simulink library "marine_hydro"  (R2019b)
settings: Solver=ode45  StartTime=0.0  StopTime=10.0  RelTol=1e-3
undefined symbols (not defined in the file): Hoerner, magnitude, slcm, vessel, vesselABC
libraries: simulink x60, marine_gnc x22, $bdroot x9
(part 2 of 4)

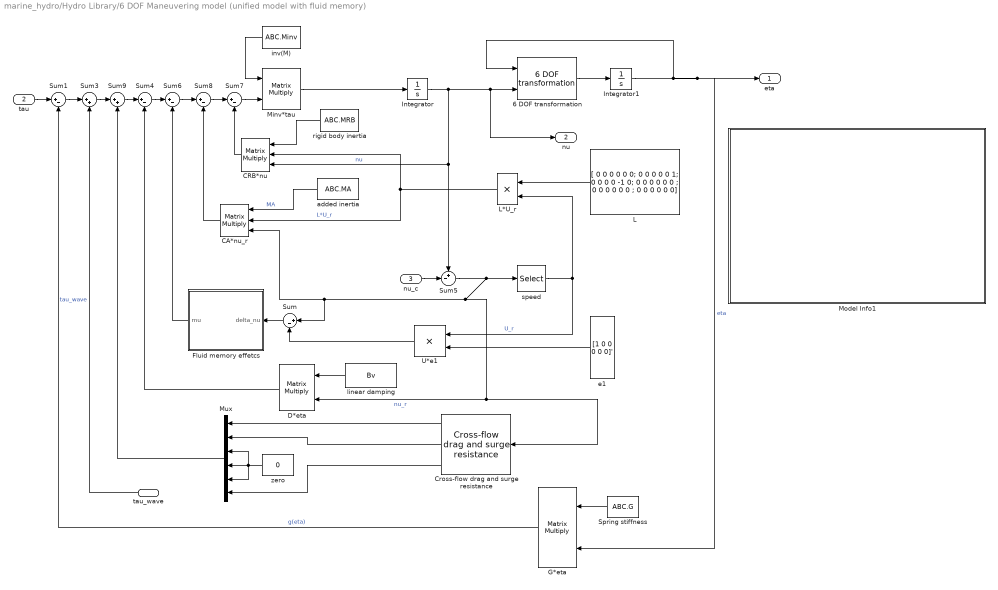
== system marine_hydro/Hydro Library/6 DOF Maneuvering model (unified model with fluid memory) ==
  tau_wave : Inport
  tau : Inport  Port=2
  nu_c : Inport  Port=3
  6 DOF transformation : marine_gnc/Models/ Kinematics/6 DOF transformation  SystemSampleTime=-1
  CA*nu_r : Product  Inputs=3  Multiplication=Matrix(*)  RndMeth=Zero
  CRB*nu : Product  Inputs=3  Multiplication=Matrix(*)  RndMeth=Zero
  Cross-flow drag and surge resistance : $bdroot/Hydro Library/Cross-flow drag and surge resistance  SystemSampleTime=-1  N=20  Lpp=vessel.main.Lpp  CD=CY_2D  Cx=CX  Ax=Axc  Ay=Ayc  rho_w=rho
  "D*eta " : Product  Multiplication=Matrix(*)  SaturateOnIntegerOverflow=on  OutDataTypeStr=Inherit: Same as first input
  Fluid memory effetcs : Subsystem
  G*eta : Product  Multiplication=Matrix(*)  SaturateOnIntegerOverflow=on  OutDataTypeStr=Inherit: Same as first input
  Integrator : Integrator
  Integrator1 : Integrator
  L : Constant  Value=|
      | [ 0     0     0     0     0     0;   0     0     0     0     0     1;
      |      0     0     0     0    -1     0;	
      |      0     0     0     0     0     0	;
      |      0     0     0     0     0     0	
      | ;     0     0     0     0     0     0]
  L*U_r : Product  RndMeth=Zero
  Minv*tau : Product  Inputs=**  Multiplication=Matrix(*)  SaturateOnIntegerOverflow=on  OutDataTypeStr=Inherit: Same as first input
  Model Info1 : Subsystem  LoadFcn=slcm LoadBlock;  InitFcn=slcm('UpdateAllCMBlocksInThisModelInit')  mask(CMBlock){InitialSaveTempField=, InitialBlockCM=None, BlockCM=None, Frame=on, SaveTempField=, DisplayStringWithTags=|, MaskDisplayString=This is an example block based on Perez and Fossen (2007).\nThe model includes speed-dependent fluid memory effects \ncross-flow drag and surge resistance (quadratic drag).\nYou must inlcude maneuvering coefficients your self. \n\nAlso notice that viscous roll damping is computed under the assumption \nof zero speed. Forward speed effects can, however, be added if necessary.\n\nReference\nT. Perez and T. I. Fossen (2007). Kinematic Models for Seakeeping\nand Maneuvering of Marine Vessels. Modeling, Identification\nand Control, MIC-28(1):1-12.\n\nDownload link: www.marinecontrol.org\n\nAuthor: Thor I. Fossen\nThu Sep 17 11:19:48 2009, HorizontalTextAlignment=Left, LeftAlignmentValue=0.02, SourceBlockDiagram=marine_hydro, TagMaxNumber=20, CMTag1=, CMTag2=, CMTag3=, CMTag4=, CMTag5=, CMTag6=, CMTag7=, CMTag8=, CMTag9=, CMTag10=, CMTag11=, CMTag12=, CMTag13=, CMTag14=, CMTag15=, CMTag16=, CMTag17=, CMTag18=, CMTag19=, CMTag20=}
      mask DisplayStringWithTags=|
      | This is an example block based on Perez and Fossen (2007).\nThe model includes speed-dependent fluid memory effects
      | cross-flow drag and surge resistance (quadratic drag).\nYou must inlcude maneuvering coefficients your self. \n
      | Also notice that viscous roll damping is computed under the assumption \nof zero speed. Forward speed effects can, however, be added if necessary.
      |
      | Reference
      | T. Perez and T. I. Fossen (2007). Kinematic Models for Seakeeping
      | and Maneuvering of Marine Vessels. Modeling, Identification\nand Control, MIC-28(1):1-12.\n
      | Download link: www.marinecontrol.org
      |
      | Author: Thor I. Fossen
      | %<LastModificationDate>
      mask help: This block allows revision control information to be displayed within the model.
      settings: CopyFcn=slcm CopyBlock;  DeleteFcn=slcm Cancel;  PostSaveFcn=slcm('UpdateAllCMBlocksInThisModel')  NameChangeFcn=slcm Rename;  OpenFcn=slcm
      mask Display: text(str2num(LeftAlignmentValue), 0.5, MaskDisplayString, 'HorizontalAlignment', HorizontalTextAlignment)
  Mux : Mux  Inputs=6
  Spring stiffness : Constant  Value=ABC.G
  Sum : Sum  Inputs=|+-
  Sum{1,4,6..8} (5 alike) : Sum  Inputs=|+-  SaturateOnIntegerOverflow=on
  Sum3 : Sum  Inputs=|++  SaturateOnIntegerOverflow=on
  Sum5 : Sum  Inputs=+-|  SaturateOnIntegerOverflow=on
  Sum9 : Sum  Inputs=|++  SaturateOnIntegerOverflow=on
  U*e1 : Product  RndMeth=Zero
  added inertia : Constant  Value=ABC.MA
  e1 : Constant  Value=[1 0 0 0 0 0]'  VectorParams1D=off
  inv(M) : Constant  Value=ABC.Minv
  linear damping : Constant  Value=Bv
  rigid body inertia : Constant  Value=ABC.MRB
  speed : Selector  InputPortWidth=6  IndexOptions=Index vector (dialog)  Indices=[1]  OutputSizes=1
  zero : Constant  Value=0
  eta : Outport
  nu : Outport  Port=2
  wires:
  speed/1 -> L*U_r/2, U*e1/1  "U_r"
  inv(M)/1 -> Minv*tau/1
  e1/1 -> U*e1/2
  U*e1/1 -> Sum/2
  Sum/1 -> Fluid memory effetcs/1(delta_nu)
  L*U_r/1 -> CA*nu_r/2, CRB*nu/2  "L*U_r"
  L/1 -> L*U_r/1
  Mux/1 -> Sum9/2
  Sum9/1 -> Sum4/1
  zero/1 -> Mux/5, Mux/3, Mux/4
  Cross-flow drag and surge resistance/3 -> Mux/6
  Cross-flow drag and surge resistance/2 -> Mux/2
  Cross-flow drag and surge resistance/1 -> Mux/1
  CA*nu_r/1 -> Sum8/2
  Sum8/1 -> Sum7/1
  CRB*nu/1 -> Sum7/2
  Fluid memory effetcs/1(mu) -> Sum6/2
  Sum7/1 -> Minv*tau/2
  Sum5/1 -> speed/1, Sum/1, CA*nu_r/3, Cross-flow drag and surge resistance/1, "D*eta "/2  "nu_r"
  nu_c/1 -> Sum5/2
  "D*eta "/1 -> Sum4/2
  linear damping/1 -> "D*eta "/1
  Integrator/1 -> CRB*nu/3, Sum5/1, nu/1, 6 DOF transformation/2  "nu"
  Sum1/1 -> Sum3/1
  Spring stiffness/1 -> G*eta/1
  added inertia/1 -> CA*nu_r/1  "MA"
  6 DOF transformation/1 -> Integrator1/1
  Integrator1/1 -> G*eta/2, eta/1, 6 DOF transformation/1  "eta"
  G*eta/1 -> Sum1/2  "g(eta)"
  rigid body inertia/1 -> CRB*nu/1
  tau/1 -> Sum1/1
  tau_wave/1 -> Sum3/2  "tau_wave"
  Sum3/1 -> Sum9/1
  Sum6/1 -> Sum8/1
  Sum4/1 -> Sum6/1
  Minv*tau/1 -> Integrator/1

== system marine_hydro/Hydro Library/Cross-flow drag and surge resistance ==
  nu_r : Inport
  "2D drag coefficient " : Constant  Value=CD
  Abs1 : Abs  SaturateOnIntegerOverflow=on
  Cross-flow drag trapezoidal integration : Subsystem  TreatAsAtomicUnit=on
  Drag coefficient : Constant  Value=Cx
  Frontal area : Constant  Value=Ax
  Gain : Gain  Gain=-0.5  SaturateOnIntegerOverflow=on  OutDataTypeStr=Inherit: Same as input  ParamDataTypeStr=Inherit: Same as input
  Gain1 : Gain  Gain=-0.5  SaturateOnIntegerOverflow=on  OutDataTypeStr=Inherit: Same as input  ParamDataTypeStr=Inherit: Same as input
  Gain2 : Gain  Gain=0.5  SaturateOnIntegerOverflow=on  OutDataTypeStr=Inherit: Same as input  ParamDataTypeStr=Inherit: Same as input
  Gain3 : Gain  Gain=-1  SaturateOnIntegerOverflow=on  OutDataTypeStr=Inherit: Same as input  ParamDataTypeStr=Inherit: Same as input
  Lpp : Constant  Value=Lpp
  N : Constant  Value=N
  Product5 : Product  Inputs=3  SaturateOnIntegerOverflow=on  OutDataTypeStr=Inherit: Same as first input
  Product7 : Product  SaturateOnIntegerOverflow=on  OutDataTypeStr=Inherit: Same as first input
  Product8 : Product  SaturateOnIntegerOverflow=on  OutDataTypeStr=Inherit: Same as first input
  Selector : Selector  InputPortWidth=6  IndexOptions=Index vector (dialog)  Indices=[2]  OutputSizes=1
  Selector1 : Selector  InputPortWidth=6  IndexOptions=Index vector (dialog)  Indices=[6]  OutputSizes=1
  Selector2 : Selector  InputPortWidth=6  IndexOptions=Index vector (dialog)  Indices=[1]  OutputSizes=1
  Sum : Sum  Inputs=+-|  SaturateOnIntegerOverflow=on  InputSameDT=on  OutDataTypeStr=Inherit: Same as first input
  Transversal area/Lpp : Constant  Value=Ay/Lpp
  constant : Constant
  dx : Product  Inputs=/*  RndMeth=Zero
  dx1 : Product  Inputs=4  RndMeth=Zero
  dx2 : Product  Inputs=4  RndMeth=Zero
  rho : Constant  Value=rho_w
  X_drag : Outport
  Y_drag : Outport  Port=2
  N_drag : Outport  Port=3
  wires:
  Product5/1 -> Product8/2
  Product7/1 -> Product8/1
  Abs1/1 -> Product7/1
  Selector2/1 -> Abs1/1, Product7/2  "u_r"
  Frontal area/1 -> Gain2/1
  Gain2/1 -> Product5/1
  "2D drag coefficient "/1 -> dx2/4, dx1/4
  Transversal area/Lpp/1 -> dx2/3, dx1/3
  N/1 -> Sum/1, Cross-flow drag trapezoidal integration/1(N)  "N"
  Sum/1 -> dx/1  "N-1"
  dx/1 -> Cross-flow drag trapezoidal integration/2(dx)
  constant/1 -> Sum/2
  Lpp/1 -> dx/2
  Selector1/1 -> Cross-flow drag trapezoidal integration/4(r)  "r"
  Selector/1 -> Cross-flow drag trapezoidal integration/3(v_r)  "v_r"
  Cross-flow drag trapezoidal integration/2(sum2) -> Gain/1
  Cross-flow drag trapezoidal integration/1(sum1) -> Gain1/1
  Gain3/1 -> X_drag/1
  Product8/1 -> Gain3/1
  nu_r/1 -> Selector2/1, Selector/1, Selector1/1
  Gain1/1 -> dx1/1
  dx1/1 -> Y_drag/1
  Gain/1 -> dx2/1
  dx2/1 -> N_drag/1
  rho/1 -> dx1/2, dx2/2, Product5/3
  Drag coefficient/1 -> Product5/2

== system marine_hydro/Hydro Library/Motion RAO (U=0) ==
  eta LF : Inport
  Waves : Inport  Port=2
  6DOF rotation matrix in yaw : Subsystem
  Bus Selector : BusSelector  OutputSignals=Psi,Wavenum,Omega,Phase,Zeta_a
  Clock : Clock
  Output smoothing : Subsystem
  Position phase : marine_gnc/Models/Environmental Loads/Utilities/Position phase  SystemSampleTime=-1
  Product1 : Product  Inputs=**  SaturateOnIntegerOverflow=on  OutDataTypeStr=Inherit: Same as first input
  Sum : Sum  Inputs=-++  SaturateOnIntegerOverflow=on
  Wave component loop : Subsystem  TreatAsAtomicUnit=on
  Width : Width  DataType=int32
  Yaw quantizer : marine_gnc/Models/Environmental Loads/Utilities/Yaw quantizer  SystemSampleTime=-1  quant_flag=RAO_yaw_quantization_flag  quant=RAO_yaw_quant  back=RAO_yaw_back
  "[-inf inf] to [-pi pi]" : marine_gnc/Utilities/Math Operations/[-inf inf] to [-pi pi]  SystemSampleTime=-1
  yaw angle : Selector  InputPortWidth=6  IndexOptions=Index vector (dialog)  Indices=6  OutputSizes=1
  eta WF : Outport
  nu WF : Outport  Port=2
  nu_dot WF : Outport  Port=3
  wires:
  Position phase/1 -> Sum/1
  "[-inf inf] to [-pi pi]"/1 -> Wave component loop/2(Psi_r)
  Yaw quantizer/1 -> "[-inf inf] to [-pi pi]"/1
  Wave component loop/3(nu_dot WF) -> Output smoothing/3("nu_dot WF ")
  Wave component loop/2(nu WF) -> Output smoothing/2("nu WF ")
  Width/1 -> Wave component loop/1(number of iterations)
  Bus Selector/5 -> Wave component loop/5(Zeta_a)  "<Zeta_a>"
  Sum/1 -> Wave component loop/4(Phase_tot)  "Phase_tot"
  6DOF rotation matrix in yaw/1(R(psi)*V) -> eta WF/1
  Bus Selector/3 -> Product1/1, Wave component loop/3(Omega), Width/1  "<Omega>"
  yaw angle/1 -> Yaw quantizer/1, 6DOF rotation matrix in yaw/1(psi)
  Clock/1 -> Product1/2
  Bus Selector/1 -> Yaw quantizer/2, Position phase/1  "<Psi>"
  Product1/1 -> Sum/2
  Waves/1 -> Bus Selector/1
  Bus Selector/4 -> Sum/3  "<Phase>"
  Bus Selector/2 -> Position phase/2  "<Wavenum>"
  eta LF/1 -> Position phase/3, yaw angle/1
  Output smoothing/2(nu WF) -> nu WF/1
  Output smoothing/3(nu_dot WF) -> nu_dot WF/1
  Wave component loop/1(eta_h WF) -> Output smoothing/1(eta_h WF)
  Wave component loop/4(nu_dot rate) -> Output smoothing/4(nu_dot rate)
  Output smoothing/1("eta_h WF ") -> 6DOF rotation matrix in yaw/2(V)

== system marine_hydro/Hydro Library/WD for heading1 ==
  psi : Inport
  psi_wave : Inport  Port=2
  Omega : Inport  Port=3
  Zeta_a : Inport  Port=4
  U : Inport  Port=5
  Sum1 : Sum  Inputs=-+|
  Wave component loop : Subsystem  TreatAsAtomicUnit=on
  Width : Width  DataType=int32
  tau_WD : Outport
  wires:
  psi/1 -> Sum1/1  "psi"
  U/1 -> Wave component loop/5(U)
  Wave component loop/1(tau_WD) -> tau_WD/1
  Sum1/1 -> Wave component loop/2(Psi_r)
  Zeta_a/1 -> Wave component loop/4(Zeta_a)
  Omega/1 -> Width/1, Wave component loop/3(Omega)
  psi_wave/1 -> Sum1/2
  Width/1 -> Wave component loop/1(number of iterations)

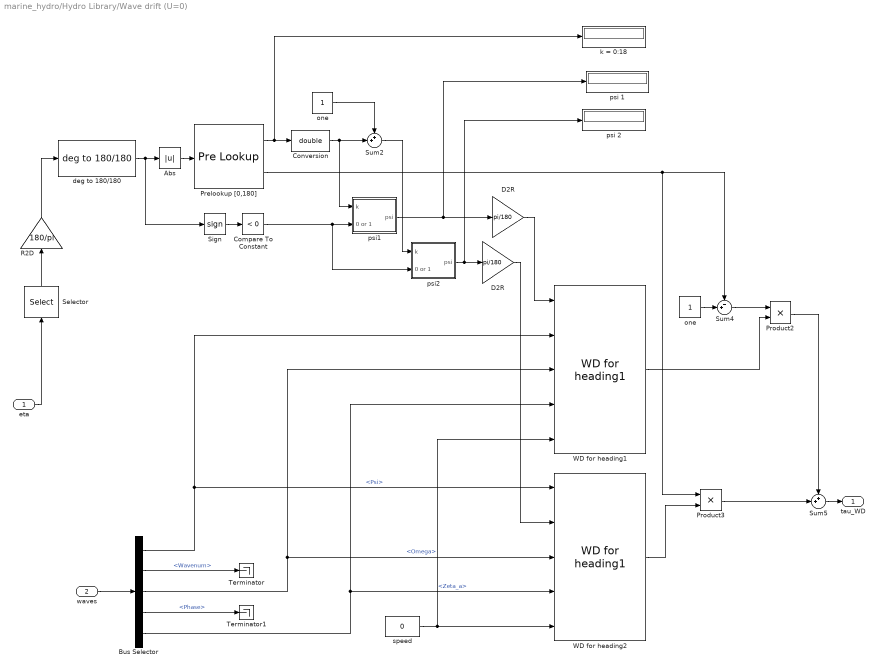
== system marine_hydro/Hydro Library/Wave drift (U=0) ==
  eta : Inport
  waves : Inport  Port=2
  Abs : Abs  SaturateOnIntegerOverflow=on
  Bus Selector : BusSelector  OutputSignals=Psi,Wavenum,Omega,Phase,Zeta_a
  Compare To Constant : simulink/Logic and Bit Operations/Compare To Constant  SystemSampleTime=-1  relop=<  const=0  LogicOutDataTypeMode=uint8  ZeroCross=off
  Conversion : DataTypeConversion  OutDataTypeStr=double
  D2R : Gain  Gain=pi/180
  "D2R " : Gain  Gain=pi/180
  Prelookup [0,180] : PreLookup  BreakpointsData=[0:10:180]  IndexSearchMethod=Evenly spaced points  BeginIndexSearchUsingPreviousIndexResult=on
  Product2 : Product  RndMeth=Zero
  Product3 : Product  RndMeth=Zero
  R2D : Gain  Gain=180/pi
  Selector : Selector  InputPortWidth=6  IndexOptions=Index vector (dialog)  Indices=[6]  OutputSizes=1
  Sign : Signum
  Sum2 : Sum  Inputs=++|
  Sum4 : Sum  Inputs=-+|
  Sum5 : Sum  Inputs=++|
  Terminator : Terminator
  Terminator1 : Terminator
  WD for heading1 : $bdroot/Hydro Library/WD for heading1  SystemSampleTime=-1  ForceRAO_Freq=vessel.forceRAO.w  WD_Freq=vessel.driftfrc.w  RAO_Vel=vessel.velocities  ForceRAO_Amp=vessel.forceRAO.amp  ForceRAO_Phase=vessel.forceRAO.phase  WD_Amp=vessel.driftfrc.amp  RAO_add_omega_0=on  RAO_add_omega_inf=on
  WD for heading2 : $bdroot/Hydro Library/WD for heading1  SystemSampleTime=-1  ForceRAO_Freq=vessel.forceRAO.w  WD_Freq=vessel.driftfrc.w  RAO_Vel=vessel.velocities  ForceRAO_Amp=vessel.forceRAO.amp  ForceRAO_Phase=vessel.forceRAO.phase  WD_Amp=vessel.driftfrc.amp  RAO_add_omega_0=on  RAO_add_omega_inf=on
  deg to 180/180 : marine_gnc/Utilities/Math Operations/deg to 180//180  SystemSampleTime=-1
  k = 0:18 : Display
  one : Constant
  "one " : Constant
  psi 1 : Display
  psi 2 : Display
  psi1 : Subsystem
  psi2 : Subsystem
  speed : Constant  Value=0
  tau_WD : Outport
  wires:
  "D2R "/1 -> WD for heading2/2
  D2R/1 -> WD for heading1/1
  Bus Selector/4 -> Terminator1/1  "<Phase>"
  Bus Selector/1 -> WD for heading2/1, WD for heading1/2  "<Psi>"
  Bus Selector/2 -> Terminator/1  "<Wavenum>"
  Bus Selector/5 -> WD for heading1/4, WD for heading2/4  "<Zeta_a>"
  Bus Selector/3 -> WD for heading1/3, WD for heading2/3  "<Omega>"
  speed/1 -> WD for heading1/5, WD for heading2/5
  R2D/1 -> deg to 180/180/1
  Selector/1 -> R2D/1
  Sum5/1 -> tau_WD/1
  waves/1 -> Bus Selector/1
  psi2/1(psi) -> psi 2/1, "D2R "/1
  Conversion/1 -> psi1/1(k), Sum2/2
  Prelookup [0,180]/2 -> Sum4/1, Product3/1
  psi1/1(psi) -> psi 1/1, D2R/1
  Compare To Constant/1 -> psi2/2(0 or 1), psi1/2(0 or 1)
  Sign/1 -> Compare To Constant/1
  Abs/1 -> Prelookup [0,180]/1
  deg to 180/180/1 -> Sign/1, Abs/1
  Sum2/1 -> psi2/1(k)
  one/1 -> Sum2/1
  Prelookup [0,180]/1 -> k = 0:18/1, Conversion/1
  Product2/1 -> Sum5/1
  Product3/1 -> Sum5/2
  WD for heading1/1 -> Product2/2
  Sum4/1 -> Product2/1
  "one "/1 -> Sum4/2
  eta/1 -> Selector/1
  WD for heading2/1 -> Product3/2

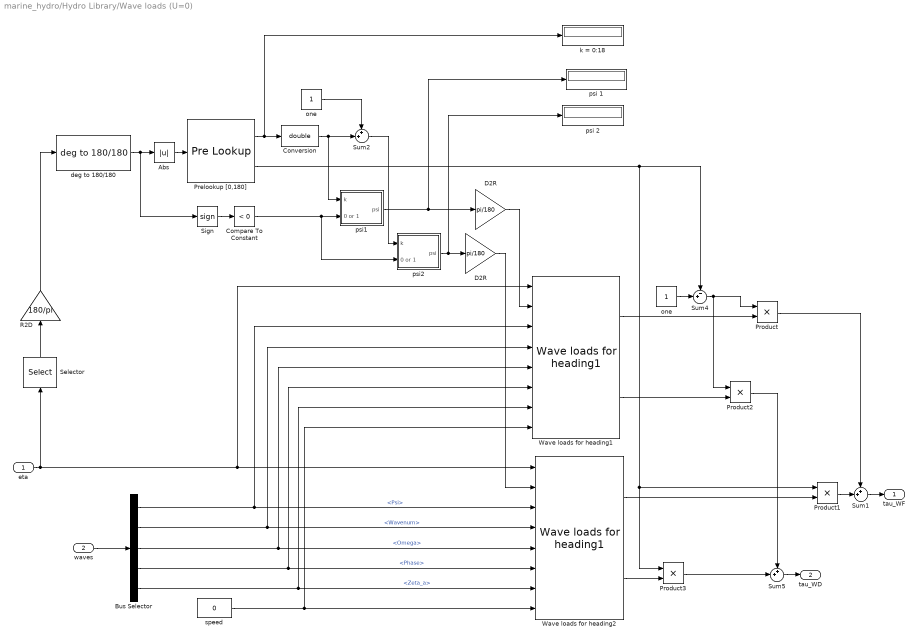
== system marine_hydro/Hydro Library/Wave loads (U=0) ==
  eta : Inport
  waves : Inport  Port=2
  Abs : Abs  SaturateOnIntegerOverflow=on
  Bus Selector : BusSelector  OutputSignals=Psi,Wavenum,Omega,Phase,Zeta_a
  Compare To Constant : simulink/Logic and Bit Operations/Compare To Constant  SystemSampleTime=-1  relop=<  const=0  LogicOutDataTypeMode=uint8  ZeroCross=off
  Conversion : DataTypeConversion  OutDataTypeStr=double
  D2R : Gain  Gain=pi/180
  "D2R " : Gain  Gain=pi/180
  Prelookup [0,180] : PreLookup  BreakpointsData=[0:10:180]  IndexSearchMethod=Evenly spaced points  BeginIndexSearchUsingPreviousIndexResult=on
  Product{,1..3} (4 alike) : Product  RndMeth=Zero
  R2D : Gain  Gain=180/pi
  Selector : Selector  InputPortWidth=6  IndexOptions=Index vector (dialog)  Indices=[6]  OutputSizes=1
  Sign : Signum
  Sum1 : Sum  Inputs=++|
  Sum2 : Sum  Inputs=++|
  Sum4 : Sum  Inputs=-+|
  Sum5 : Sum  Inputs=++|
  Wave loads for heading1 : $bdroot/Hydro Library/Wave loads for heading1  SystemSampleTime=-1  ForceRAO_Freq=vessel.forceRAO.w  WD_Freq=vessel.driftfrc.w  RAO_Vel=vessel.velocities  ForceRAO_Amp=vessel.forceRAO.amp  ForceRAO_Phase=vessel.forceRAO.phase  WD_Amp=vessel.driftfrc.amp  RAO_add_omega_0=on  RAO_add_omega_inf=on
  Wave loads for heading2 : $bdroot/Hydro Library/Wave loads for heading1  SystemSampleTime=-1  ForceRAO_Freq=vessel.forceRAO.w  WD_Freq=vessel.driftfrc.w  RAO_Vel=vessel.velocities  ForceRAO_Amp=vessel.forceRAO.amp  ForceRAO_Phase=vessel.forceRAO.phase  WD_Amp=vessel.driftfrc.amp  RAO_add_omega_0=on  RAO_add_omega_inf=on
  deg to 180/180 : marine_gnc/Utilities/Math Operations/deg to 180//180  SystemSampleTime=-1
  k = 0:18 : Display
  one : Constant
  "one " : Constant
  psi 1 : Display
  psi 2 : Display
  psi1 : Subsystem
  psi2 : Subsystem
  speed : Constant  Value=0
  tau_WF : Outport
  tau_WD : Outport  Port=2
  wires:
  speed/1 -> Wave loads for heading1/8, Wave loads for heading2/8
  Wave loads for heading2/1 -> Product1/2
  Wave loads for heading2/2 -> Product3/2
  eta/1 -> Wave loads for heading1/1, Wave loads for heading2/1, Selector/1
  Bus Selector/1 -> Wave loads for heading1/3, Wave loads for heading2/3  "<Psi>"
  Bus Selector/2 -> Wave loads for heading1/4, Wave loads for heading2/4  "<Wavenum>"
  Bus Selector/3 -> Wave loads for heading1/5, Wave loads for heading2/5  "<Omega>"
  Bus Selector/4 -> Wave loads for heading1/6, Wave loads for heading2/6  "<Phase>"
  Bus Selector/5 -> Wave loads for heading1/7, Wave loads for heading2/7  "<Zeta_a>"
  Wave loads for heading1/1 -> Product/2
  Product/1 -> Sum1/1
  Product1/1 -> Sum1/2
  "one "/1 -> Sum4/2
  Sum4/1 -> Product/1, Product2/1
  Wave loads for heading1/2 -> Product2/2
  Product3/1 -> Sum5/2
  Product2/1 -> Sum5/1
  Prelookup [0,180]/1 -> Conversion/1, k = 0:18/1
  one/1 -> Sum2/1
  Sum2/1 -> psi2/1(k)
  deg to 180/180/1 -> Abs/1, Sign/1
  Abs/1 -> Prelookup [0,180]/1
  Sign/1 -> Compare To Constant/1
  Compare To Constant/1 -> psi1/2(0 or 1), psi2/2(0 or 1)
  psi1/1(psi) -> D2R/1, psi 1/1
  Prelookup [0,180]/2 -> Product3/1, Product1/1, Sum4/1
  Conversion/1 -> Sum2/2, psi1/1(k)
  psi2/1(psi) -> "D2R "/1, psi 2/1
  D2R/1 -> Wave loads for heading1/2
  "D2R "/1 -> Wave loads for heading2/2
  Sum1/1 -> tau_WF/1
  waves/1 -> Bus Selector/1
  Sum5/1 -> tau_WD/1
  Selector/1 -> R2D/1
  R2D/1 -> deg to 180/180/1

== system marine_hydro/Hydro Library/Wave loads (U>0) ==
  eta : Inport
  waves : Inport  Port=2
  U : Inport  Port=3
  Abs : Abs  SaturateOnIntegerOverflow=on
  Conversion : DataTypeConversion  OutDataTypeStr=double
  Prelookup : PreLookup  BreakpointsData=vessel.velocities  IndexSearchMethod=Linear search  BeginIndexSearchUsingPreviousIndexResult=on
  Product{,1..3} (4 alike) : Product  RndMeth=Zero
  Sum1 : Sum  Inputs=++|
  Sum2 : Sum  Inputs=++|
  Sum4 : Sum  Inputs=-+|
  Sum5 : Sum  Inputs=++|
  Wave loads U = U1 : Subsystem
  Wave loads U = U2 : Subsystem
  one : Constant
  "one " : Constant
  tau_WF : Outport
  tau_WD : Outport  Port=2
  wires:
  waves/1 -> Wave loads U = U1/2(waves), Wave loads U = U2/2(waves)
  eta/1 -> Wave loads U = U1/1(eta), Wave loads U = U2/1(eta)
  Conversion/1 -> Sum2/2, Wave loads U = U1/3(U_idx)
  Abs/1 -> Prelookup/1
  one/1 -> Sum2/1
  Prelookup/1 -> Conversion/1
  Sum2/1 -> Wave loads U = U2/3(U_idx)
  Sum5/1 -> tau_WD/1
  Sum1/1 -> tau_WF/1
  Prelookup/2 -> Sum4/1, Product1/1, Product3/1
  Product2/1 -> Sum5/1
  Product3/1 -> Sum5/2
  Sum4/1 -> Product2/1, Product/1
  "one "/1 -> Sum4/2
  Product1/1 -> Sum1/2
  Product/1 -> Sum1/1
  Wave loads U = U1/1(tau_WF) -> Product/2
  Wave loads U = U2/2(tau_WD) -> Product3/2
  Wave loads U = U2/1(tau_WF) -> Product1/2
  Wave loads U = U1/2(tau_WD) -> Product2/2
  U/1 -> Abs/1

== system marine_hydro/Hydro Library/Wave loads for heading1 ==
  eta : Inport
  psi : Inport  Port=2
  psi_wave : Inport  Port=3
  wavenum : Inport  Port=4
  Omega : Inport  Port=5
  Phase : Inport  Port=6
  Zeta_a : Inport  Port=7
  U : Inport  Port=8
  Clock : Clock
  Position phase : marine_gnc/Models/Environmental Loads/Utilities/Position phase  SystemSampleTime=-1
  Product1 : Product  Inputs=**  SaturateOnIntegerOverflow=on  OutDataTypeStr=Inherit: Same as first input
  Sum : Sum  Inputs=-++  SaturateOnIntegerOverflow=on
  Sum1 : Sum  Inputs=-+|
  Wave component loop : Subsystem  TreatAsAtomicUnit=on
  Width : Width  DataType=int32
  tau_WF : Outport
  tau_WD : Outport  Port=2
  wires:
  Position phase/1 -> Sum/1
  Width/1 -> Wave component loop/1(number of iterations)
  Sum/1 -> Wave component loop/4(Phase_tot)  "Phase_tot"
  Clock/1 -> Product1/2
  Product1/1 -> Sum/2
  Wave component loop/1(tau_WF) -> tau_WF/1
  eta/1 -> Position phase/3
  psi_wave/1 -> Position phase/1, Sum1/2
  wavenum/1 -> Position phase/2
  Omega/1 -> Product1/1, Wave component loop/3(Omega), Width/1
  Phase/1 -> Sum/3
  Zeta_a/1 -> Wave component loop/5(Zeta_a)
  Sum1/1 -> Wave component loop/2(Psi_r)
  Wave component loop/2(tau_WD) -> tau_WD/1
  U/1 -> Wave component loop/6(U)
  psi/1 -> Sum1/1  "psi"

== system marine_hydro/Hydro Library/zero speed viiscous roll damping ==
  p : Inport
  A44 : Constant  Value=vesselABC.A44(:,:,1)
  B44 : Constant  Value=vesselABC.B44(:,:,1)
  B44_inf : Constant  Value=vesselABC.B44_inf(1)
  C44 : Constant  Value=vesselABC.C44(:,:,1)
  D44 : Constant  Value=vesselABC.D44(:,:,1)
  Integrator : Integrator
  Math Function : Math  Operator=transpose  SaturateOnIntegerOverflow=on
  Product{,1..2,4} (4 alike) : Product  Multiplication=Matrix(*)  RndMeth=Zero
  Product3 : Product  RndMeth=Zero
  Sum : Sum  Inputs=++|
  Sum1 : Sum  Inputs=|++
  Sum2 : Sum  Inputs=++|
  K_visc : Outport
  wires:
  Product4/1 -> Sum2/1
  B44_inf/1 -> Product4/1
  Sum2/1 -> K_visc/1
  p/1 -> Product4/2, Product1/2, Product3/2
  Integrator/1 -> Product/2, Product2/2
  A44/1 -> Product/1
  Product1/1 -> Sum/1
  Product/1 -> Sum/2
  Sum/1 -> Integrator/1
  C44/1 -> Math Function/1
  D44/1 -> Product3/1
  Product3/1 -> Sum1/2
  Product2/1 -> Sum1/1
  Sum1/1 -> Sum2/2
  B44/1 -> Product1/1
  Math Function/1 -> Product2/1

== system marine_hydro/Vessel Templates/DP Force RAO model - zero speed ==
  Gain : Gain  SaturateOnIntegerOverflow=on  OutDataTypeStr=Inherit: Same as input  ParamDataTypeStr=Inherit: Same as input

== system marine_hydro/Vessel Templates/DP Motion RAO model - zero speed ==
  Gain : Gain  SaturateOnIntegerOverflow=on  OutDataTypeStr=Inherit: Same as input  ParamDataTypeStr=Inherit: Same as input

== system marine_hydro/Vessel Templates/Maneuvering Force RAO model - forward speed ==
  Gain : Gain  SaturateOnIntegerOverflow=on  OutDataTypeStr=Inherit: Same as input  ParamDataTypeStr=Inherit: Same as input

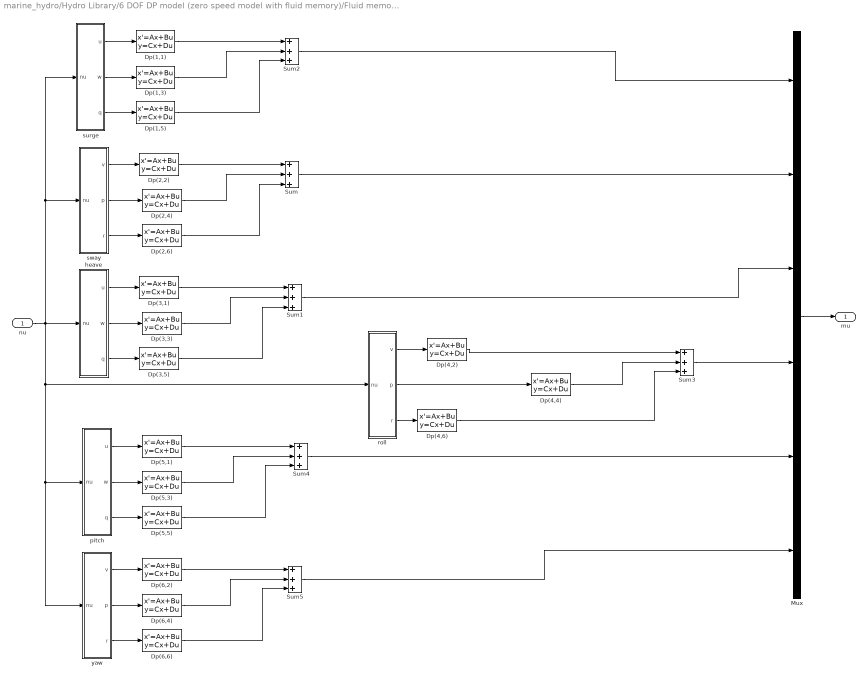
== system marine_hydro/Hydro Library/6 DOF DP model (zero speed model with fluid memory)/Fluid memory effetcs ==
  nu : Inport
  Dp(1,1) : StateSpace  A=ABC.Ar{1,1}  B=ABC.Br{1,1}  C=ABC.Cr{1,1}  D=ABC.Dr{1,1}  InitialCondition=0
  Dp(1,3) : StateSpace  A=ABC.Ar{1,3}  B=ABC.Br{1,3}  C=ABC.Cr{1,3}  D=ABC.Dr{1,3}  InitialCondition=0
  Dp(1,5) : StateSpace  A=ABC.Ar{1,5}  B=ABC.Br{1,5}  C=ABC.Cr{1,5}  D=ABC.Dr{1,5}  InitialCondition=0
  Dp(2,2) : StateSpace  A=ABC.Ar{2,2}  B=ABC.Br{2,2}  C=ABC.Cr{2,2}  D=ABC.Dr{2,2}  InitialCondition=0
  Dp(2,4) : StateSpace  A=ABC.Ar{2,4}  B=ABC.Br{2,4}  C=ABC.Cr{2,4}  D=ABC.Dr{2,4}  InitialCondition=0
  Dp(2,6) : StateSpace  A=ABC.Ar{2,6}  B=ABC.Br{2,6}  C=ABC.Cr{2,6}  D=ABC.Dr{2,6}  InitialCondition=0
  Dp(3,1) : StateSpace  A=ABC.Ar{3,1}  B=ABC.Br{3,1}  C=ABC.Cr{3,1}  D=ABC.Dr{3,1}  InitialCondition=0
  Dp(3,3) : StateSpace  A=ABC.Ar{3,3}  B=ABC.Br{3,3}  C=ABC.Cr{3,3}  D=ABC.Dr{3,3}  InitialCondition=0
  Dp(3,5) : StateSpace  A=ABC.Ar{3,5}  B=ABC.Br{3,5}  C=ABC.Cr{3,5}  D=ABC.Dr{3,5}  InitialCondition=0
  Dp(4,2) : StateSpace  A=ABC.Ar{4,2}  B=ABC.Br{4,2}  C=ABC.Cr{4,2}  D=ABC.Dr{4,2}  InitialCondition=0
  Dp(4,4) : StateSpace  A=ABC.Ar{4,4}  B=ABC.Br{4,4}  C=ABC.Cr{4,4}  D=ABC.Dr{4,4}  InitialCondition=0
  Dp(4,6) : StateSpace  A=ABC.Ar{4,6}  B=ABC.Br{4,6}  C=ABC.Cr{4,6}  D=ABC.Dr{4,6}  InitialCondition=0
  Dp(5,1) : StateSpace  A=ABC.Ar{5,1}  B=ABC.Br{5,1}  C=ABC.Cr{5,1}  D=ABC.Dr{5,1}  InitialCondition=0
  Dp(5,3) : StateSpace  A=ABC.Ar{5,3}  B=ABC.Br{5,3}  C=ABC.Cr{5,3}  D=ABC.Dr{5,3}  InitialCondition=0
  Dp(5,5) : StateSpace  A=ABC.Ar{5,5}  B=ABC.Br{5,5}  C=ABC.Cr{5,5}  D=ABC.Dr{5,5}  InitialCondition=0
  Dp(6,2) : StateSpace  A=ABC.Ar{6,2}  B=ABC.Br{6,2}  C=ABC.Cr{6,2}  D=ABC.Dr{6,2}  InitialCondition=0
  Dp(6,4) : StateSpace  A=ABC.Ar{6,4}  B=ABC.Br{6,4}  C=ABC.Cr{6,4}  D=ABC.Dr{6,4}  InitialCondition=0
  Dp(6,6) : StateSpace  A=ABC.Ar{6,6}  B=ABC.Br{6,6}  C=ABC.Cr{6,6}  D=ABC.Dr{6,6}  InitialCondition=0
  Mux : Mux  Inputs=6
  Sum{,1..5} (6 alike) : Sum  Inputs=+++  SaturateOnIntegerOverflow=on
  heave : Subsystem
  pitch : Subsystem
  roll : Subsystem
  surge : Subsystem
  sway : Subsystem
  yaw : Subsystem
  mu : Outport
  wires:
  Sum4/1 -> Mux/5
  Dp(2,2)/1 -> Sum/1
  Dp(2,4)/1 -> Sum/2
  Dp(2,6)/1 -> Sum/3
  Sum/1 -> Mux/2
  sway/1(v) -> Dp(2,2)/1
  sway/2(p) -> Dp(2,4)/1
  sway/3(r) -> Dp(2,6)/1
  Dp(3,3)/1 -> Sum1/2
  Dp(3,5)/1 -> Sum1/3
  Sum1/1 -> Mux/3
  heave/3(q) -> Dp(3,5)/1
  heave/2(w) -> Dp(3,3)/1
  heave/1(u) -> Dp(3,1)/1
  Dp(3,1)/1 -> Sum1/1
  nu/1 -> heave/1(nu), sway/1(nu), surge/1(nu), roll/1(nu), pitch/1(nu), yaw/1(nu)
  Mux/1 -> mu/1
  Dp(1,3)/1 -> Sum2/2
  Dp(1,5)/1 -> Sum2/3
  Sum2/1 -> Mux/1
  surge/3(q) -> Dp(1,5)/1
  surge/2(w) -> Dp(1,3)/1
  surge/1(u) -> Dp(1,1)/1
  Dp(1,1)/1 -> Sum2/1
  Dp(4,2)/1 -> Sum3/1
  Dp(4,6)/1 -> Sum3/3
  roll/1(v) -> Dp(4,2)/1
  roll/3(r) -> Dp(4,6)/1
  Dp(5,3)/1 -> Sum4/2
  Dp(5,5)/1 -> Sum4/3
  pitch/3(q) -> Dp(5,5)/1
  pitch/2(w) -> Dp(5,3)/1
  pitch/1(u) -> Dp(5,1)/1
  Dp(5,1)/1 -> Sum4/1
  Sum3/1 -> Mux/4
  Dp(6,2)/1 -> Sum5/1
  Dp(6,4)/1 -> Sum5/2
  Dp(6,6)/1 -> Sum5/3
  yaw/1(v) -> Dp(6,2)/1
  yaw/2(p) -> Dp(6,4)/1
  yaw/3(r) -> Dp(6,6)/1
  Sum5/1 -> Mux/6
  roll/2(p) -> Dp(4,4)/1
  Dp(4,4)/1 -> Sum3/2

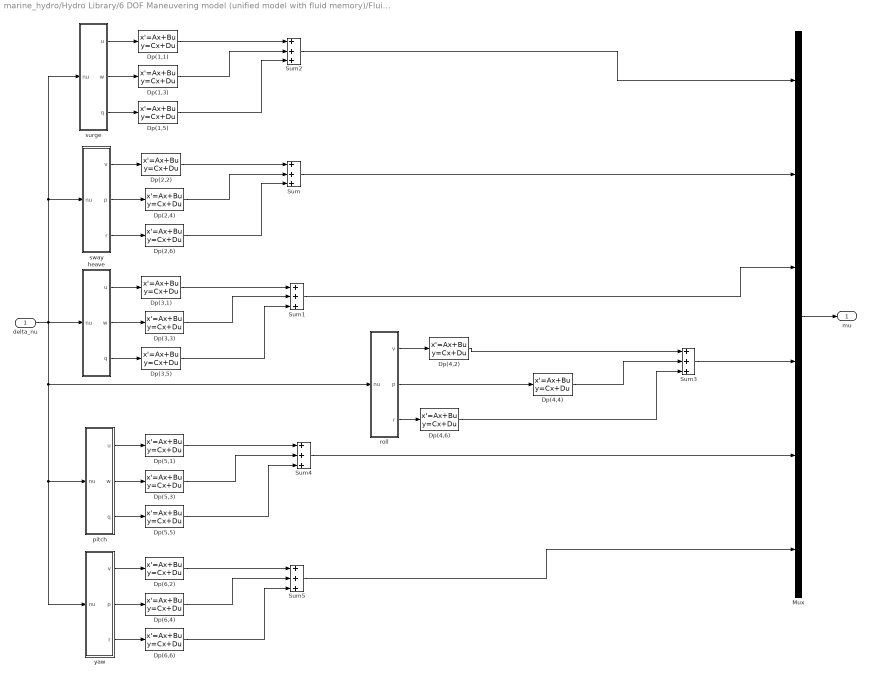
== system marine_hydro/Hydro Library/6 DOF Maneuvering model (unified model with fluid memory)/Fluid memory effetcs ==
  delta_nu : Inport
  Dp(1,1) : StateSpace  A=ABC.Ar{1,1}  B=ABC.Br{1,1}  C=ABC.Cr{1,1}  D=ABC.Dr{1,1}  InitialCondition=0
  Dp(1,3) : StateSpace  A=ABC.Ar{1,3}  B=ABC.Br{1,3}  C=ABC.Cr{1,3}  D=ABC.Dr{1,3}  InitialCondition=0
  Dp(1,5) : StateSpace  A=ABC.Ar{1,5}  B=ABC.Br{1,5}  C=ABC.Cr{1,5}  D=ABC.Dr{1,5}  InitialCondition=0
  Dp(2,2) : StateSpace  A=ABC.Ar{2,2}  B=ABC.Br{2,2}  C=ABC.Cr{2,2}  D=ABC.Dr{2,2}  InitialCondition=0
  Dp(2,4) : StateSpace  A=ABC.Ar{2,4}  B=ABC.Br{2,4}  C=ABC.Cr{2,4}  D=ABC.Dr{2,4}  InitialCondition=0
  Dp(2,6) : StateSpace  A=ABC.Ar{2,6}  B=ABC.Br{2,6}  C=ABC.Cr{2,6}  D=ABC.Dr{2,6}  InitialCondition=0
  Dp(3,1) : StateSpace  A=ABC.Ar{3,1}  B=ABC.Br{3,1}  C=ABC.Cr{3,1}  D=ABC.Dr{3,1}  InitialCondition=0
  Dp(3,3) : StateSpace  A=ABC.Ar{3,3}  B=ABC.Br{3,3}  C=ABC.Cr{3,3}  D=ABC.Dr{3,3}  InitialCondition=0
  Dp(3,5) : StateSpace  A=ABC.Ar{3,5}  B=ABC.Br{3,5}  C=ABC.Cr{3,5}  D=ABC.Dr{3,5}  InitialCondition=0
  Dp(4,2) : StateSpace  A=ABC.Ar{4,2}  B=ABC.Br{4,2}  C=ABC.Cr{4,2}  D=ABC.Dr{4,2}  InitialCondition=0
  Dp(4,4) : StateSpace  A=ABC.Ar{4,4}  B=ABC.Br{4,4}  C=ABC.Cr{4,4}  D=ABC.Dr{4,4}  InitialCondition=0
  Dp(4,6) : StateSpace  A=ABC.Ar{4,6}  B=ABC.Br{4,6}  C=ABC.Cr{4,6}  D=ABC.Dr{4,6}  InitialCondition=0
  Dp(5,1) : StateSpace  A=ABC.Ar{5,1}  B=ABC.Br{5,1}  C=ABC.Cr{5,1}  D=ABC.Dr{5,1}  InitialCondition=0
  Dp(5,3) : StateSpace  A=ABC.Ar{5,3}  B=ABC.Br{5,3}  C=ABC.Cr{5,3}  D=ABC.Dr{5,3}  InitialCondition=0
  Dp(5,5) : StateSpace  A=ABC.Ar{5,5}  B=ABC.Br{5,5}  C=ABC.Cr{5,5}  D=ABC.Dr{5,5}  InitialCondition=0
  Dp(6,2) : StateSpace  A=ABC.Ar{6,2}  B=ABC.Br{6,2}  C=ABC.Cr{6,2}  D=ABC.Dr{6,2}  InitialCondition=0
  Dp(6,4) : StateSpace  A=ABC.Ar{6,4}  B=ABC.Br{6,4}  C=ABC.Cr{6,4}  D=ABC.Dr{6,4}  InitialCondition=0
  Dp(6,6) : StateSpace  A=ABC.Ar{6,6}  B=ABC.Br{6,6}  C=ABC.Cr{6,6}  D=ABC.Dr{6,6}  InitialCondition=0
  Mux : Mux  Inputs=6
  Sum{,1..5} (6 alike) : Sum  Inputs=+++  SaturateOnIntegerOverflow=on
  heave : Subsystem
  pitch : Subsystem
  roll : Subsystem
  surge : Subsystem
  sway : Subsystem
  yaw : Subsystem
  mu : Outport
  wires:
  Sum4/1 -> Mux/5
  Dp(2,2)/1 -> Sum/1
  Dp(2,4)/1 -> Sum/2
  Dp(2,6)/1 -> Sum/3
  Sum/1 -> Mux/2
  sway/1(v) -> Dp(2,2)/1
  sway/2(p) -> Dp(2,4)/1
  sway/3(r) -> Dp(2,6)/1
  Dp(3,3)/1 -> Sum1/2
  Dp(3,5)/1 -> Sum1/3
  Sum1/1 -> Mux/3
  heave/3(q) -> Dp(3,5)/1
  heave/2(w) -> Dp(3,3)/1
  heave/1(u) -> Dp(3,1)/1
  Dp(3,1)/1 -> Sum1/1
  delta_nu/1 -> heave/1(nu), sway/1(nu), surge/1(nu), roll/1(nu), pitch/1(nu), yaw/1(nu)
  Mux/1 -> mu/1
  Dp(1,3)/1 -> Sum2/2
  Dp(1,5)/1 -> Sum2/3
  Sum2/1 -> Mux/1
  surge/3(q) -> Dp(1,5)/1
  surge/2(w) -> Dp(1,3)/1
  surge/1(u) -> Dp(1,1)/1
  Dp(1,1)/1 -> Sum2/1
  Dp(4,2)/1 -> Sum3/1
  Dp(4,6)/1 -> Sum3/3
  roll/1(v) -> Dp(4,2)/1
  roll/3(r) -> Dp(4,6)/1
  Dp(5,3)/1 -> Sum4/2
  Dp(5,5)/1 -> Sum4/3
  pitch/3(q) -> Dp(5,5)/1
  pitch/2(w) -> Dp(5,3)/1
  pitch/1(u) -> Dp(5,1)/1
  Dp(5,1)/1 -> Sum4/1
  Sum3/1 -> Mux/4
  Dp(6,2)/1 -> Sum5/1
  Dp(6,4)/1 -> Sum5/2
  Dp(6,6)/1 -> Sum5/3
  yaw/1(v) -> Dp(6,2)/1
  yaw/2(p) -> Dp(6,4)/1
  yaw/3(r) -> Dp(6,6)/1
  Sum5/1 -> Mux/6
  roll/2(p) -> Dp(4,4)/1
  Dp(4,4)/1 -> Sum3/2

== system marine_hydro/Hydro Library/6 DOF Maneuvering model (unified model with fluid memory)/Model Info1 ==
  EmptySubsystem : Subsystem

== system marine_hydro/Hydro Library/Cross-flow drag and surge resistance/Cross-flow drag trapezoidal integration ==
  N : Inport
  dx : Inport  Port=2
  v_r : Inport  Port=3
  r : Inport  Port=4
  Abs : Abs  SaturateOnIntegerOverflow=on
  For Iterator : ForIterator  ResetStates=reset  IterationSource=external  IterationVariableDataType=double
  If i=1 or i=N : If  NumInputs=2  IfExpression=u1 == 1 | u1 == u2
  Lpp/2 : Constant  Value=Lpp/2
  Merge : Merge
  Product : Product  Inputs=**  SaturateOnIntegerOverflow=on  OutDataTypeStr=Inherit: Same as first input
  Product1 : Product  Inputs=**  SaturateOnIntegerOverflow=on  OutDataTypeStr=Inherit: Same as first input
  Product3 : Product  SaturateOnIntegerOverflow=on  OutDataTypeStr=Inherit: Same as first input
  Product4 : Product  SaturateOnIntegerOverflow=on  OutDataTypeStr=Inherit: Same as first input
  Sum : Sum  Inputs=|++  SaturateOnIntegerOverflow=on  InputSameDT=on  OutDataTypeStr=Inherit: Same as first input
  Sum1 : Sum  Inputs=++|  SaturateOnIntegerOverflow=on
  Sum2 : Sum  Inputs=|++  SaturateOnIntegerOverflow=on  InputSameDT=on  OutDataTypeStr=Inherit: Same as first input
  Sum3 : Sum  Inputs=+-|  SaturateOnIntegerOverflow=on  InputSameDT=on  OutDataTypeStr=Inherit: Same as first input
  Sum4 : Sum  Inputs=+-|  SaturateOnIntegerOverflow=on  InputSameDT=on  OutDataTypeStr=Inherit: Same as first input
  constant : Constant
  memory1 : Memory  InheritSampleTime=on
  memory2 : Memory  InheritSampleTime=on
  multiply with 0.5 : Subsystem  TreatAsAtomicUnit=on
  multiply with 1 : Subsystem  TreatAsAtomicUnit=on
  x * r : Product  SaturateOnIntegerOverflow=on  OutDataTypeStr=Inherit: Same as first input
  sum1 : Outport
  sum2 : Outport  Port=2
  wires:
  Merge/1 -> Product4/1, Sum/2
  multiply with 1/1(Out1) -> Merge/2
  multiply with 0.5/1(Out1) -> Merge/1
  If i=1 or i=N/2 -> multiply with 1/Action
  If i=1 or i=N/1 -> multiply with 0.5/Action
  Product/1 -> multiply with 0.5/1(In1), multiply with 1/1(In1)
  Product3/1 -> Product/2
  Product4/1 -> Sum2/2
  r/1 -> x * r/1
  Sum3/1 -> Product4/2, x * r/2  "x"
  constant/1 -> Sum4/2
  Sum4/1 -> Product1/2  "i-1"
  Product1/1 -> Sum3/1
  Lpp/2/1 -> Sum3/2
  dx/1 -> Product/1, Product1/1  "dx"
  memory2/1 -> Sum2/1
  Sum2/1 -> memory2/1, sum2/1
  memory1/1 -> Sum/1
  Sum/1 -> memory1/1, sum1/1
  v_r/1 -> Sum1/1
  Abs/1 -> Product3/1
  x * r/1 -> Sum1/2
  Sum1/1 -> Abs/1, Product3/2
  N/1 -> If i=1 or i=N/2, For Iterator/1
  For Iterator/1 -> Sum4/1, If i=1 or i=N/1  "i"

== system marine_hydro/Hydro Library/Motion RAO (U=0)/6DOF rotation matrix in yaw ==
  psi : Inport
  V : Inport  Port=2
  Mux1 : Mux  Inputs=2
  Rotation matrix in yaw : marine_gnc/Models/ Kinematics/Rotation matrix in yaw   SystemSampleTime=-1
  Selector : Selector  InputPortWidth=6  IndexOptions=Index vector (dialog)  Indices=[4 5 6]  OutputSizes=1
  Selector2 : Selector  InputPortWidth=6  IndexOptions=Index vector (dialog)  Indices=[1 2 3]  OutputSizes=1
  R(psi)*V : Outport
  wires:
  Selector/1 -> Mux1/2
  Mux1/1 -> R(psi)*V/1
  Selector2/1 -> Rotation matrix in yaw/2
  psi/1 -> Rotation matrix in yaw/1
  V/1 -> Selector2/1, Selector/1
  Rotation matrix in yaw/1 -> Mux1/1

== system marine_hydro/Hydro Library/Motion RAO (U=0)/Output smoothing ==
  eta_h WF : Inport
  "nu WF " : Inport  Port=2
  "nu_dot WF " : Inport  Port=3
  nu_dot rate : Inport  Port=4
  Output smoothing flag : Constant  Value=RAO_smoothing_flag
  Signal smoothing : marine_gnc/Models/Environmental Loads/Utilities/Signal smoothing  SystemSampleTime=-1
  Signal smoothing1 : marine_gnc/Models/Environmental Loads/Utilities/Signal smoothing  SystemSampleTime=-1
  Signal smoothing2 : marine_gnc/Models/Environmental Loads/Utilities/Signal smoothing  SystemSampleTime=-1
  Switch1 : Switch  Threshold=0.5
  Switch2 : Switch  Threshold=0.5
  Switch3 : Switch  Threshold=0.5
  "eta_h WF " : Outport
  nu WF : Outport  Port=2
  nu_dot WF : Outport  Port=3
  wires:
  Output smoothing flag/1 -> Switch2/2, Switch1/2, Switch3/2
  Signal smoothing/1 -> Switch2/1
  eta_h WF/1 -> Signal smoothing/1, Switch2/3
  "nu WF "/1 -> Signal smoothing1/1, Signal smoothing/2, Switch1/3
  Signal smoothing1/1 -> Switch1/1
  Switch2/1 -> "eta_h WF "/1
  "nu_dot WF "/1 -> Signal smoothing2/1, Signal smoothing1/2, Switch3/3
  Signal smoothing2/1 -> Switch3/1
  nu_dot rate/1 -> Signal smoothing2/2
  Switch3/1 -> nu_dot WF/1
  Switch1/1 -> nu WF/1

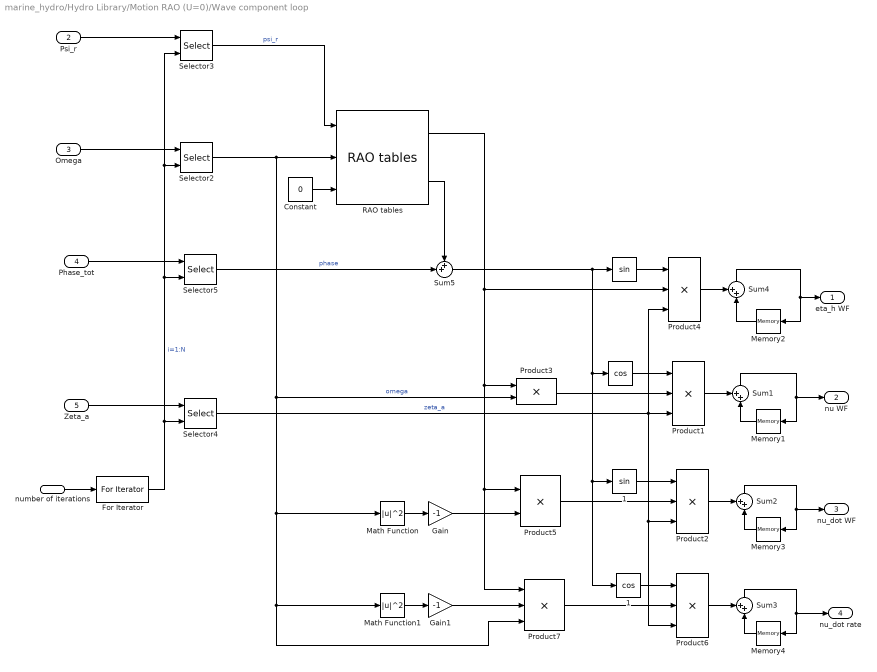
== system marine_hydro/Hydro Library/Motion RAO (U=0)/Wave component loop ==
  number of iterations : Inport
  Psi_r : Inport  Port=2
  Omega : Inport  Port=3
  Phase_tot : Inport  Port=4
  Zeta_a : Inport  Port=5
  "              " : Trigonometry  Operator=cos
  "                " : Trigonometry
  "                1" : Trigonometry
  "              1" : Trigonometry  Operator=cos
  Constant : Constant  Value=0
  For Iterator : ForIterator  ResetStates=reset  IterationSource=external  IterationVariableDataType=double
  Gain : Gain  Gain=-1  SaturateOnIntegerOverflow=on  OutDataTypeStr=Inherit: Same as input  ParamDataTypeStr=Inherit: Same as input
  Gain1 : Gain  Gain=-1  SaturateOnIntegerOverflow=on  OutDataTypeStr=Inherit: Same as input  ParamDataTypeStr=Inherit: Same as input
  Math Function : Math  Operator=magnitude^2  SaturateOnIntegerOverflow=on
  Math Function1 : Math  Operator=magnitude^2  SaturateOnIntegerOverflow=on
  Memory{1..4} (4 alike) : Memory  InitialCondition=[0 0 0 0 0 0]'  InheritSampleTime=on
  Product{1..2,4,6} (4 alike) : Product  Inputs=3  SaturateOnIntegerOverflow=on  OutDataTypeStr=Inherit: Same as first input
  Product3 : Product  Inputs=**  SaturateOnIntegerOverflow=on  OutDataTypeStr=Inherit: Same as first input
  Product5 : Product  Inputs=**  SaturateOnIntegerOverflow=on  OutDataTypeStr=Inherit: Same as first input
  Product7 : Product  Inputs=***  SaturateOnIntegerOverflow=on  OutDataTypeStr=Inherit: Same as first input
  RAO tables : marine_gnc/Models/Environmental Loads/Utilities/RAO tables  SystemSampleTime=-1  RAO_Freq=RAO_Freq  RAO_Dir=RAO_Dir  RAO_Vel=RAO_Vel  RAO_Amp=RAO_Amp  RAO_Phase=RAO_Phase
  Selector{2..5} (4 alike) : Selector  IndexOptions=Index vector (port)  Indices=[1 3]  OutputSizes=1
  Sum{1..5} (5 alike) : Sum  Inputs=++|  SaturateOnIntegerOverflow=on
  eta_h WF : Outport
  nu WF : Outport  Port=2
  nu_dot WF : Outport  Port=3
  nu_dot rate : Outport  Port=4
  wires:
  Product3/1 -> Product1/2
  Product5/1 -> Product2/2
  Gain/1 -> Product5/2
  Math Function/1 -> Gain/1
  "                1"/1 -> Product2/1
  Sum2/1 -> Memory3/1, nu_dot WF/1
  Product2/1 -> Sum2/1
  Memory3/1 -> Sum2/2
  Product1/1 -> Sum1/1
  Sum1/1 -> Memory1/1, nu WF/1
  Memory1/1 -> Sum1/2
  "              "/1 -> Product1/1
  Selector4/1 -> Product4/3, Product1/3, Product2/3, Product6/3  "zeta_a"
  "                "/1 -> Product4/1
  Sum5/1 -> "              "/1, "                1"/1, "              1"/1, "                "/1
  Zeta_a/1 -> Selector4/1
  Phase_tot/1 -> Selector5/1
  RAO tables/2 -> Sum5/1
  RAO tables/1 -> Product3/1, Product5/1, Product7/1, Product4/2
  Constant/1 -> RAO tables/3
  Psi_r/1 -> Selector3/1
  For Iterator/1 -> Selector4/2, Selector5/2, Selector2/2, Selector3/2  "i=1:N"
  Omega/1 -> Selector2/1
  number of iterations/1 -> For Iterator/1
  Sum4/1 -> Memory2/1, eta_h WF/1
  Memory2/1 -> Sum4/2
  Product4/1 -> Sum4/1
  Selector5/1 -> Sum5/2  "phase"
  Selector2/1 -> RAO tables/2, Product3/2, Math Function/1, Math Function1/1, Product7/3  "omega"
  Selector3/1 -> RAO tables/1  "psi_r"
  Sum3/1 -> nu_dot rate/1, Memory4/1
  Product6/1 -> Sum3/1
  Memory4/1 -> Sum3/2
  Gain1/1 -> Product7/2
  Math Function1/1 -> Gain1/1
  "              1"/1 -> Product6/1
  Product7/1 -> Product6/2

== system marine_hydro/Hydro Library/WD for heading1/Wave component loop ==
  number of iterations : Inport
  Psi_r : Inport  Port=2
  Omega : Inport  Port=3
  Zeta_a : Inport  Port=4
  U : Inport  Port=5
  Direct Lookup Table (n-D) Beta : simulink/Lookup Tables/Direct Lookup Table (n-D)  maskTabDims=1  explicitNumDims=1  outDims=Element  tabIsInput=off  mxTable=vessel.headings  clipFlag=Warning  samptime=-1
      settings: SourceProductName=Simulink  SourceProductBaseCode=SL
  Direct Lookup Table (n-D) Velocity : simulink/Lookup Tables/Direct Lookup Table (n-D)  maskTabDims=1  explicitNumDims=1  outDims=Element  tabIsInput=off  mxTable=RAO_Vel  clipFlag=Warning  samptime=-1
      settings: SourceProductName=Simulink  SourceProductBaseCode=SL
  For Iterator : ForIterator  ResetStates=reset  IterationSource=external  IterationVariableDataType=double
  Memory1 : Memory  InitialCondition=[0 0 0 0 0 0]'  InheritSampleTime=on
  Prelookup1 : PreLookup  BreakpointsData=vessel.headings  OutputSelection=Index only  IndexSearchMethod=Evenly spaced points  BeginIndexSearchUsingPreviousIndexResult=on
  Prelookup2 : PreLookup  BreakpointsData=RAO_Vel  OutputSelection=Index only  IndexSearchMethod=Linear search  BeginIndexSearchUsingPreviousIndexResult=on
  Product3 : Product  Inputs=3  SaturateOnIntegerOverflow=on  OutDataTypeStr=Inherit: Same as first input
  Selector2 : Selector  IndexOptions=Index vector (port)  Indices=[1 3]  OutputSizes=1
  Selector3 : Selector  IndexOptions=Index vector (port)  Indices=[1 3]  OutputSizes=1
  Selector4 : Selector  IndexOptions=Index vector (port)  Indices=[1 3]  OutputSizes=1
  Sum1 : Sum  Inputs=++|  SaturateOnIntegerOverflow=on
  WD RAO tables : Subsystem  mask(RAO table lookup){}
      mask help:
      | Perform 3D table lookup in 6DOF RAO amplitudes and phases, using the relative wave heading psi_r, wave frequency omega and vessel velocity vel as inputs. See documentation of the Motion RAO block or Force RAO block for details. A warning is issued if the input is outside the range spanned by the RAOs.
      |
      | Author: Oyvind N. Smogeli and Thor I. Fossen, 2005-05-03
  "[-inf inf] to [-pi pi]" : marine_gnc/Utilities/Math Operations/[-inf inf] to [-pi pi]  SystemSampleTime=-1
  "[-pi pi] to [0 2pi]" : Subsystem  mask([-inf inf] to [-pi pi]){}
      mask help: Converts an angle in rad to (-pi pi)
  tau_WD : Outport
  wires:
  WD RAO tables/1(amp) -> Product3/1
  Direct Lookup Table (n-D) Velocity/1 -> WD RAO tables/3(U)
  Prelookup2/1 -> Direct Lookup Table (n-D) Velocity/1
  Direct Lookup Table (n-D) Beta/1 -> WD RAO tables/1(beta)
  Prelookup1/1 -> Direct Lookup Table (n-D) Beta/1
  "[-inf inf] to [-pi pi]"/1 -> "[-pi pi] to [0 2pi]"/1(x [-pi pi])
  For Iterator/1 -> Selector2/2, Selector4/2, Selector3/2  "i=1:N"
  Selector2/1 -> WD RAO tables/2(w)  "omega"
  "[-pi pi] to [0 2pi]"/1(0<y<2pi) -> Prelookup1/1
  Product3/1 -> Sum1/1
  Memory1/1 -> Sum1/2
  Sum1/1 -> tau_WD/1, Memory1/1
  Selector3/1 -> "[-inf inf] to [-pi pi]"/1  "psi_r"
  number of iterations/1 -> For Iterator/1
  Omega/1 -> Selector2/1
  Psi_r/1 -> Selector3/1
  U/1 -> Prelookup2/1
  Zeta_a/1 -> Selector4/1
  Selector4/1 -> Product3/3, Product3/2  "zeta_a"

== system marine_hydro/Hydro Library/Wave drift (U=0)/psi1 ==
  k : Inport
  0 or 1 : Inport  Port=2
  Gain1 : Gain  Gain=20
  Gain2 : Gain  Gain=10
  Product : Product  RndMeth=Zero
  Sum7 : Sum  Inputs=-+|
  Sum8 : Sum  Inputs=++|
  const : Constant  Value=18
  psi : Outport
  wires:
  0 or 1/1 -> Product/2
  Sum8/1 -> psi/1
  k/1 -> Gain2/1, Sum7/1
  Gain2/1 -> Sum8/1
  Product/1 -> Sum8/2
  Gain1/1 -> Product/1
  Sum7/1 -> Gain1/1
  const/1 -> Sum7/2

== system marine_hydro/Hydro Library/Wave drift (U=0)/psi2 ==
  k : Inport
  0 or 1 : Inport  Port=2
  Gain1 : Gain  Gain=20
  Gain2 : Gain  Gain=10
  Product : Product  RndMeth=Zero
  Sum7 : Sum  Inputs=-+|
  Sum8 : Sum  Inputs=++|
  const : Constant  Value=18
  psi : Outport
  wires:
  0 or 1/1 -> Product/2
  Sum8/1 -> psi/1
  k/1 -> Gain2/1, Sum7/1
  Gain2/1 -> Sum8/1
  Product/1 -> Sum8/2
  Gain1/1 -> Product/1
  Sum7/1 -> Gain1/1
  const/1 -> Sum7/2

== system marine_hydro/Hydro Library/Wave loads (U=0)/psi1 ==
  k : Inport
  0 or 1 : Inport  Port=2
  Gain1 : Gain  Gain=20
  Gain2 : Gain  Gain=10
  Product : Product  RndMeth=Zero
  Sum7 : Sum  Inputs=-+|
  Sum8 : Sum  Inputs=++|
  const : Constant  Value=18
  psi : Outport
  wires:
  const/1 -> Sum7/2
  Sum7/1 -> Gain1/1
  Gain1/1 -> Product/1
  Product/1 -> Sum8/2
  Gain2/1 -> Sum8/1
  k/1 -> Sum7/1, Gain2/1
  Sum8/1 -> psi/1
  0 or 1/1 -> Product/2

== system marine_hydro/Hydro Library/Wave loads (U=0)/psi2 ==
  k : Inport
  0 or 1 : Inport  Port=2
  Gain1 : Gain  Gain=20
  Gain2 : Gain  Gain=10
  Product : Product  RndMeth=Zero
  Sum7 : Sum  Inputs=-+|
  Sum8 : Sum  Inputs=++|
  const : Constant  Value=18
  psi : Outport
  wires:
  const/1 -> Sum7/2
  Sum7/1 -> Gain1/1
  Gain1/1 -> Product/1
  Product/1 -> Sum8/2
  Gain2/1 -> Sum8/1
  k/1 -> Sum7/1, Gain2/1
  Sum8/1 -> psi/1
  0 or 1/1 -> Product/2

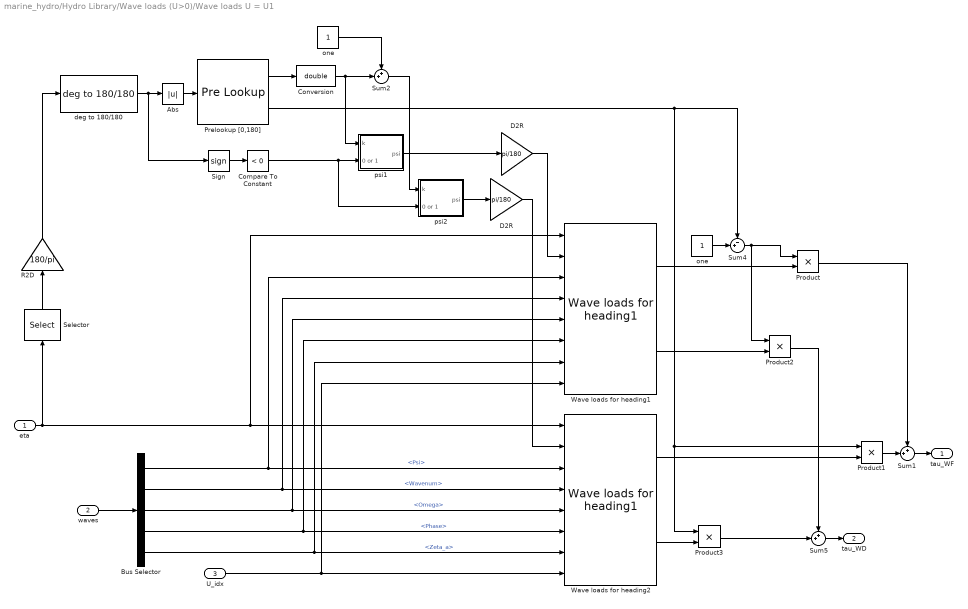
== system marine_hydro/Hydro Library/Wave loads (U>0)/Wave loads U = U1 ==
  eta : Inport
  waves : Inport  Port=2
  U_idx : Inport  Port=3
  Abs : Abs  SaturateOnIntegerOverflow=on
  Bus Selector : BusSelector  OutputSignals=Psi,Wavenum,Omega,Phase,Zeta_a
  Compare To Constant : simulink/Logic and Bit Operations/Compare To Constant  SystemSampleTime=-1  relop=<  const=0  LogicOutDataTypeMode=uint8  ZeroCross=off
  Conversion : DataTypeConversion  OutDataTypeStr=double
  D2R : Gain  Gain=pi/180
  "D2R " : Gain  Gain=pi/180
  Prelookup [0,180] : PreLookup  BreakpointsData=[0:10:180]  IndexSearchMethod=Evenly spaced points  BeginIndexSearchUsingPreviousIndexResult=on
  Product{,1..3} (4 alike) : Product  RndMeth=Zero
  R2D : Gain  Gain=180/pi
  Selector : Selector  InputPortWidth=6  IndexOptions=Index vector (dialog)  Indices=[6]  OutputSizes=1
  Sign : Signum
  Sum1 : Sum  Inputs=++|
  Sum2 : Sum  Inputs=++|
  Sum4 : Sum  Inputs=-+|
  Sum5 : Sum  Inputs=++|
  Wave loads for heading1 : $bdroot/Hydro Library/Wave loads for heading1  SystemSampleTime=-1  ForceRAO_Freq=vessel.forceRAO.w  WD_Freq=vessel.driftfrc.w  RAO_Vel=vessel.velocities  ForceRAO_Amp=vessel.forceRAO.amp  ForceRAO_Phase=vessel.forceRAO.phase  WD_Amp=vessel.driftfrc.amp  RAO_add_omega_0=on  RAO_add_omega_inf=on
  Wave loads for heading2 : $bdroot/Hydro Library/Wave loads for heading1  SystemSampleTime=-1  ForceRAO_Freq=vessel.forceRAO.w  WD_Freq=vessel.driftfrc.w  RAO_Vel=vessel.velocities  ForceRAO_Amp=vessel.forceRAO.amp  ForceRAO_Phase=vessel.forceRAO.phase  WD_Amp=vessel.driftfrc.amp  RAO_add_omega_0=on  RAO_add_omega_inf=on
  deg to 180/180 : marine_gnc/Utilities/Math Operations/deg to 180//180  SystemSampleTime=-1
  one : Constant
  "one " : Constant
  psi1 : Subsystem
  psi2 : Subsystem
  tau_WF : Outport
  tau_WD : Outport  Port=2
  wires:
  R2D/1 -> deg to 180/180/1
  Selector/1 -> R2D/1
  Sum5/1 -> tau_WD/1
  waves/1 -> Bus Selector/1
  Sum1/1 -> tau_WF/1
  "D2R "/1 -> Wave loads for heading2/2
  D2R/1 -> Wave loads for heading1/2
  psi2/1(psi) -> "D2R "/1
  Conversion/1 -> psi1/1(k), Sum2/2
  Prelookup [0,180]/2 -> Sum4/1, Product1/1, Product3/1
  psi1/1(psi) -> D2R/1
  Compare To Constant/1 -> psi2/2(0 or 1), psi1/2(0 or 1)
  Sign/1 -> Compare To Constant/1
  Abs/1 -> Prelookup [0,180]/1
  deg to 180/180/1 -> Sign/1, Abs/1
  Sum2/1 -> psi2/1(k)
  one/1 -> Sum2/1
  Prelookup [0,180]/1 -> Conversion/1
  Product2/1 -> Sum5/1
  Product3/1 -> Sum5/2
  Wave loads for heading1/2 -> Product2/2
  Sum4/1 -> Product2/1, Product/1
  "one "/1 -> Sum4/2
  Product1/1 -> Sum1/2
  Product/1 -> Sum1/1
  Wave loads for heading1/1 -> Product/2
  Bus Selector/5 -> Wave loads for heading1/7, Wave loads for heading2/7  "<Zeta_a>"
  Bus Selector/4 -> Wave loads for heading1/6, Wave loads for heading2/6  "<Phase>"
  Bus Selector/3 -> Wave loads for heading1/5, Wave loads for heading2/5  "<Omega>"
  Bus Selector/2 -> Wave loads for heading1/4, Wave loads for heading2/4  "<Wavenum>"
  Bus Selector/1 -> Wave loads for heading1/3, Wave loads for heading2/3  "<Psi>"
  eta/1 -> Selector/1, Wave loads for heading1/1, Wave loads for heading2/1
  Wave loads for heading2/2 -> Product3/2
  Wave loads for heading2/1 -> Product1/2
  U_idx/1 -> Wave loads for heading1/8, Wave loads for heading2/8
